simulink model "PIDcontroller"  (R2025b)
settings: Solver=VariableStepAuto  StartTime=0.0  StopTime=20.0  RelTol=1e-3
settings Model: Creator=ASUS  LastModifiedBy=ASUS

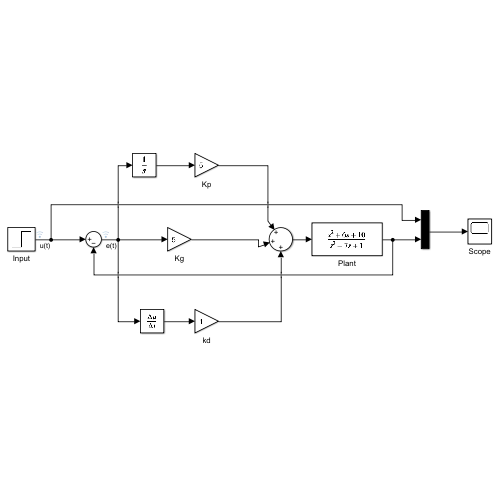
[thumbnail: Simulink's stored preview of the top-level diagram]
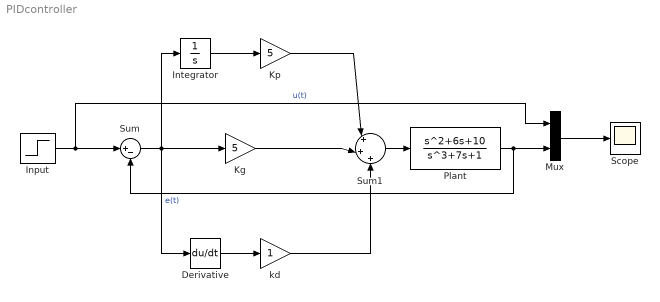
== system PIDcontroller ==
  Derivative : Derivative
  Input : Step  Tag=Imput  SampleTime=0
  Integrator : Integrator
  Kg : Gain  Gain=5
  Kp : Gain  Gain=5
  Mux : Mux  Inputs=2
  Plant : TransferFcn  Numerator=[1 6 10]  Denominator=[1 0 7 1]
  Scope : Scope
      settings: ActiveDisplayYMinimum=-1.3229523173939084  ActiveDisplayYMaximum=2.5702433677026288
  Sum : Sum  Inputs=|+-
  Sum1 : Sum  Inputs=|+|+|+
  kd : Gain
  wires:
  Plant/1 -> Mux/2, Sum/2
  Sum/1 -> Derivative/1, Integrator/1, Kg/1  "e(t)"
  Integrator/1 -> Kp/1
  Derivative/1 -> kd/1
  Sum1/1 -> Plant/1
  Kg/1 -> Sum1/2
  Kp/1 -> Sum1/1
  kd/1 -> Sum1/3
  Input/1 -> Mux/1, Sum/1  "u(t)"
  Mux/1 -> Scope/1
